simulink model "assignment2_group12"  (R2021a)
settings: Solver=FixedStepAuto  StartTime=0.0  StopTime=10.0  FixedStep=1e-3  RelTol=1e-3  EnableMultiTasking=on
undefined symbols (not defined in the file): A0, A1, D0, D1, D10, D11, D12, D13, D2, D3, D4, D5, D6, D7, D8, D9, PTA0, PTA1, PTA2, PTB2, PTB23, PTB3, PTB9, PTC16, PTC17, PTC2, PTC3, PTC4, PTD0, PTD1, PTD2, PTD3
libraries: frdmk64flib x19, etargetslib x18, dspstat3 x1
settings Model: ExtModeTrigDuration=5  Creator=shoghisama  LastModifiedBy=shoghisama
settings OptimizationCC: EnhancedBackFolding=on  PassReuseOutputArgsAs=Individual arguments  ZeroExternalMemoryAtStartup=off  ZeroInternalMemoryAtStartup=off  MaxStackSize=64  OptimizeBlockOrder=speed  DifferentSizesBufferReuse=on  OptimizationCustomize=off  EfficientTunableParamExpr=on
settings DebuggingCC: ParameterTunabilityLossMsg=error
settings HardwareCC: ProdBitPerPointer=32  ProdBitPerSizeT=32  ProdBitPerPtrDiffT=32  ProdLargestAtomicInteger=Long  ProdLargestAtomicFloat=Double  ProdWordSize=32  ProdHWDeviceType=ARM Compatible->ARM Cortex
settings SFSimCC: MATLABDynamicMemAlloc=off
settings RTWCC: SystemTargetFile=ert.tlc  HardwareBoard=NXP FRDM-K64F  TLCOptions="-aInlineSetEventsForThisBaseRateFcn=TLC_FALSE -aSuppressMultiTaskScheduler=TLC_FALSE  -aRateBasedStepFcn=0"  TemplateMakefile=ert_default_tmf  Toolchain=GNU Tools for ARM Embedded Processors
settings CodeAppCC: ForceParamTrailComments=on  IgnoreCustomStorageClasses=off  OperatorAnnotations=on  SimulinkDataObjDesc=on  SFDataObjDesc=on  InsertBlockDesc=on
settings ERTTargetCC: ExtModeTransport=4  ExtModeMexFile=sendToCommService

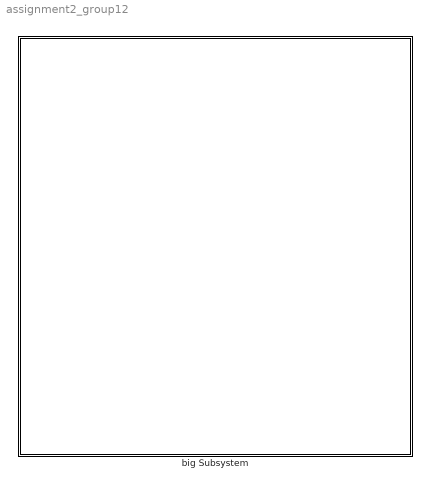
== system assignment2_group12 ==
  big Subsystem : Subsystem

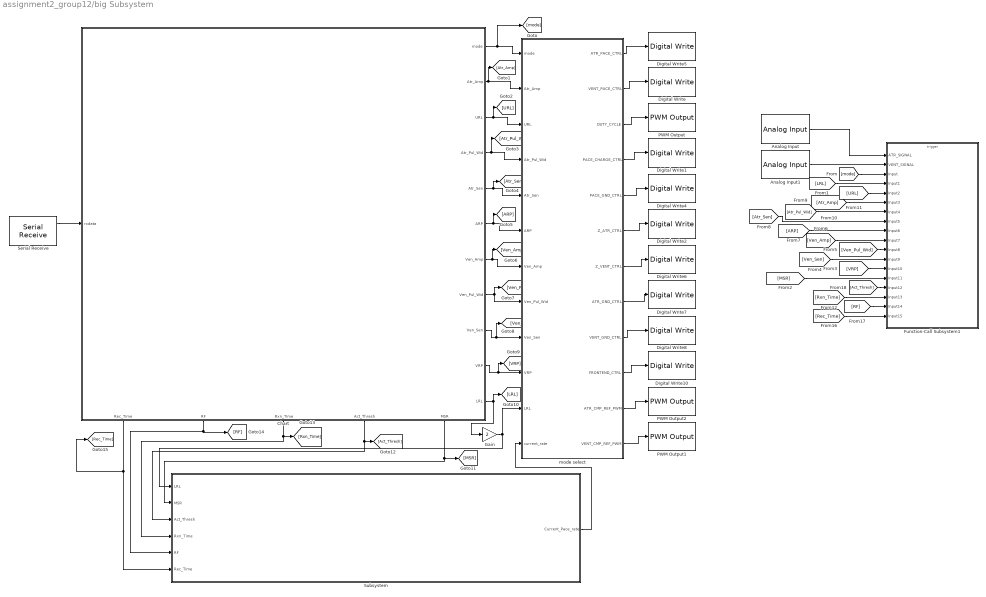
== system assignment2_group12/big Subsystem ==
  Analog Input : frdmk64flib/Analog Input  Whichpin=PTB2 (A0)  SampleTime=-1
  Analog Input1 : frdmk64flib/Analog Input  Whichpin=PTB3 (A1)  SampleTime=-1
  Chart : Stateflow chart  TreatAsAtomicUnit=on
      settings: PortSchema="{\"entries\":[{\"content\":{\"sides\":[{\"content\":{\"connectorIds\":[\"In1\"]},\"type\":\"ConnectorPlacement.EquallySpacedRectSide\",\"uuid\":\"029204fe-544c-471c-b678-20eb9ec2f0de\"},{\"content\":{\"connectorIds\":[\"Out16\",\"Out2\",\"Out3\",\"Out4\",\"Out5\",\"Out6\",\"Out7\",\"Out8\",\"Out9\",\"Out10\",\"Out1\"],\"side\":\"RIGHT\"},\"type\":\"ConnectorPlacement.EquallySpacedRectSide\",\"uuid\":\"7eca2d38-9628-43b8-9613-7fbfe5c4b303\"},{\"content\":{\"connectorIds\":[],\"side\":\"TOP\"},\"type\":\"ConnectorPlacement.EquallySpacedRectSide\",\"uuid\":\"096b792e-b126-4483-96fc-02dd5bb2fe66\"},{\"content\":{\"connectorIds\":[\"Out15\",\"Out14\",\"Out13\",\"Out12\",\"Out11\"],\"side\":\"BOTTOM\"},\"type\":\"ConnectorPlacement.EquallySpacedRectSide\",\"uuid\":\"986cb6f9-09d3-4d0e-abe9-ddef6787962a\"}]},\"type\":\"ConnectorPlacement.EquallySpacedConnector\",\"uuid\":\"f90ba696-ad08-4385-b69c-5e6e3d9fa11d\"}],\"packageUris\":[\"http://schema.mathworks.com/mf0/Connector/R2020b\"],\"version\":\"1.0\"}"
  Digital Write : frdmk64flib/Digital Write  Whichpin=PTC4 (D9)
  Digital Write1 : frdmk64flib/Digital Write  Whichpin=PTB9 (D2)
  Digital Write10 : frdmk64flib/Digital Write  Whichpin=PTD1 (D13)
  Digital Write2 : frdmk64flib/Digital Write  Whichpin=PTB23 (D4)
  Digital Write4 : frdmk64flib/Digital Write  Whichpin=PTD0 (D10)
  Digital Write5 : frdmk64flib/Digital Write  Whichpin=PTA0 (D8)
  Digital Write6 : frdmk64flib/Digital Write  Whichpin=PTC3 (D7)
  Digital Write7 : frdmk64flib/Digital Write  Whichpin=PTD2 (D11)
  Digital Write8 : frdmk64flib/Digital Write  Whichpin=PTD3 (D12)
  Function-Call Subsystem1 : Subsystem  TreatAsAtomicUnit=on
  Gain : Gain  Gain=2  OutDataTypeStr=double
  PWM Output : frdmk64flib/PWM Output  Whichpin=PTA2 (D5)  InitialFrequency=2000  InitialDutyCycle=0
  PWM Output1 : frdmk64flib/PWM Output  Whichpin=PTA1 (D3)  InitialFrequency=2000  InitialDutyCycle=0
  PWM Output2 : frdmk64flib/PWM Output  Whichpin=PTC2 (D6)  InitialFrequency=2000  InitialDutyCycle=0
  Serial Receive : frdmk64flib/Serial Receive  SCIModule=0  Baudrate=uint32(9600)  Parity=None  StopBits=1  HardwareFlowControl=None  ByteOrder=LittleEndian  DataType=uint8  DataLength=123  BlockingMode=off  OutputStatus=on  SampleTime=-1
  Subsystem : Subsystem
  mode select : Subsystem
  wires:
  Chart/4(Atr_Pul_Wid) -> [Atr_Pul_Wid], mode select/4(Atr_Pul_Wid)
  Chart/5(Atr_Sen) -> [Atr_Sen], mode select/5(Atr_Sen)
  mode select/8(ATR_GND_CTRL) -> Digital Write7/1
  mode select/4(PACE_CHARGE_CTRL) -> Digital Write1/1
  mode select/1(ATR_PACE_CTRL) -> Digital Write5/1
  mode select/2(VENT_PACE_CTRL) -> Digital Write/1
  mode select/5(PACE_GND_CTRL) -> Digital Write4/1
  mode select/6(Z_ATR_CTRL) -> Digital Write2/1
  mode select/10(FRONTEND_CTRL) -> Digital Write10/1
  mode select/7(Z_VENT_CTRL) -> Digital Write6/1
  mode select/3(DUTY_CYCLE) -> PWM Output/1
  mode select/9(VENT_GND_CTRL) -> Digital Write8/1
  mode select/12(VENT_CMP_REF_PWM) -> PWM Output1/1
  mode select/11(ATR_CMP_REF_PWM) -> PWM Output2/1
  Chart/2(Atr_Amp) -> mode select/2(Atr_Amp), [Atr_Amp]
  Chart/11(MSR) -> [MSR], Subsystem/2(MSR)
  Chart/12(Act_Thresh) -> [Act_Thresh], Subsystem/3(Act_Thresh)
  Chart/13(Rxn_Time) -> Subsystem/4(Rxn_Time), [Rxn_Time]
  Chart/14(RF) -> [RF], Subsystem/5(RF)
  Chart/15(Rec_Time) -> [Rec_Time], Subsystem/6(Rec_Time)
  Serial Receive/1 -> Chart/1(rxdata)
  Chart/6(ARP) -> [ARP], mode select/6(ARP)
  Chart/7(Ven_Amp) -> [Ven_Amp], mode select/7(Ven_Amp)
  Chart/10(VRP) -> [VRP], mode select/10(VRP)
  Chart/9(Ven_Sen) -> [Ven_Sen], mode select/9(Ven_Sen)
  Chart/8(Ven_Pul_Wid) -> mode select/8(Ven_Pul_Wid), [Ven_Pul_Wid]
  Chart/3(URL) -> [URL], mode select/3(URL)
  Subsystem/1(Current_Pace_rate) -> mode select/12(current_rate)
  Gain/1 -> mode select/11(LRL), Subsystem/1(LRL)
  Chart/16(mode) -> [mode], mode select/1(mode)
  Chart/1(LRL) -> Gain/1, [LRL]
  [ARP] -> Function-Call Subsystem1/9(Input6)
  [Rec_Time] -> Function-Call Subsystem1/18(Input15)
  [Ven_Pul_Wid] -> Function-Call Subsystem1/11(Input8)
  [URL] -> Function-Call Subsystem1/5(Input2)
  Analog Input/1 -> Function-Call Subsystem1/1(ATR_SIGNAL)
  [Atr_Sen] -> Function-Call Subsystem1/8(Input5)
  [VRP] -> Function-Call Subsystem1/13(Input10)
  [Ven_Sen] -> Function-Call Subsystem1/12(Input9)
  [LRL] -> Function-Call Subsystem1/4(Input1)
  [MSR] -> Function-Call Subsystem1/14(Input11)
  [Ven_Amp] -> Function-Call Subsystem1/10(Input7)
  [Atr_Pul_Wid] -> Function-Call Subsystem1/7(Input4)
  Analog Input1/1 -> Function-Call Subsystem1/2(VENT_SIGNAL)
  [Rxn_Time] -> Function-Call Subsystem1/16(Input13)
  [RF] -> Function-Call Subsystem1/17(Input14)
  [mode] -> Function-Call Subsystem1/3(Input)
  [Atr_Amp] -> Function-Call Subsystem1/6(Input3)
  [Act_Thresh] -> Function-Call Subsystem1/15(Input12)

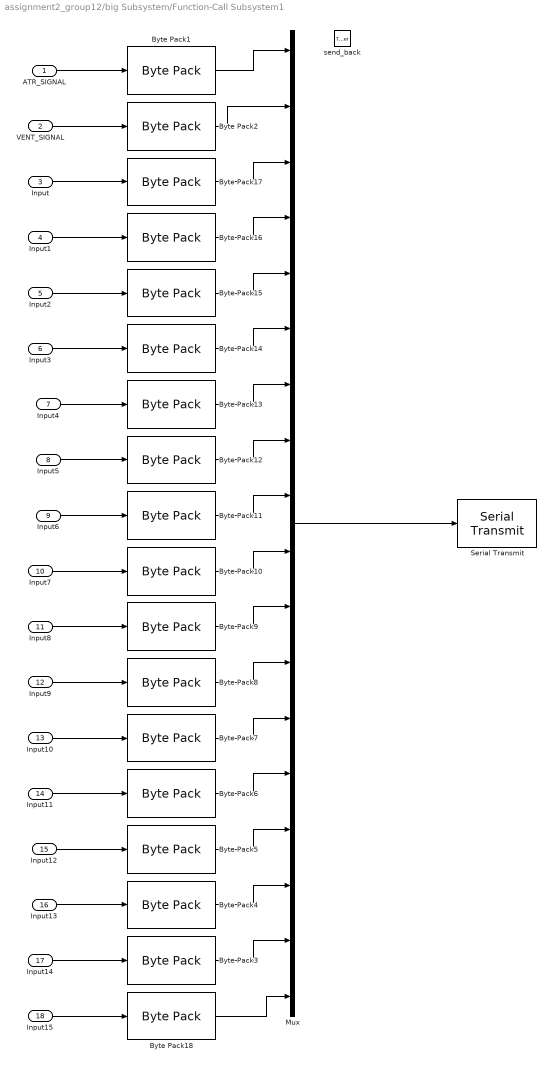
== system assignment2_group12/big Subsystem/Function-Call Subsystem1 ==
  ATR_SIGNAL : Inport  OutDataTypeStr=double
  VENT_SIGNAL : Inport  Port=2  OutDataTypeStr=double
  Input : Inport  Port=3
  Input1 : Inport  Port=4
  Input2 : Inport  Port=5
  Input3 : Inport  Port=6
  Input4 : Inport  Port=7
  Input5 : Inport  Port=8
  Input6 : Inport  Port=9
  Input7 : Inport  Port=10
  Input8 : Inport  Port=11
  Input9 : Inport  Port=12
  Input10 : Inport  Port=13
  Input11 : Inport  Port=14
  Input12 : Inport  Port=15
  Input13 : Inport  Port=16
  Input14 : Inport  Port=17
  Input15 : Inport  Port=18
  send_back : TriggerPort  TriggerType=function-call  IsSimulinkFunction=on  FunctionName=send_back  VariantControl=Variant
  Byte Pack{1..16,18} (17 alike) : etargetslib/Byte Pack  datatypes={'double'}  byteAlign=1
  Byte Pack17 : etargetslib/Byte Pack  datatypes={'uint8'}  byteAlign=1
  Mux : Mux  Inputs=18
  Serial Transmit : frdmk64flib/Serial Transmit  SCIModule=0  Baudrate=uint32(9600)  Parity=None  StopBits=1  HardwareFlowControl=None  ByteOrder=LittleEndian  BlockingMode=on  OutputStatus=off
  wires:
  Mux/1 -> Serial Transmit/1
  ATR_SIGNAL/1 -> Byte Pack1/1
  Byte Pack1/1 -> Mux/1
  VENT_SIGNAL/1 -> Byte Pack2/1
  Byte Pack2/1 -> Mux/2
  Input/1 -> Byte Pack17/1
  Input1/1 -> Byte Pack16/1
  Input2/1 -> Byte Pack15/1
  Input3/1 -> Byte Pack14/1
  Input4/1 -> Byte Pack13/1
  Input5/1 -> Byte Pack12/1
  Input6/1 -> Byte Pack11/1
  Input7/1 -> Byte Pack10/1
  Input8/1 -> Byte Pack9/1
  Input9/1 -> Byte Pack8/1
  Input13/1 -> Byte Pack4/1
  Input14/1 -> Byte Pack3/1
  Input12/1 -> Byte Pack5/1
  Input11/1 -> Byte Pack6/1
  Input10/1 -> Byte Pack7/1
  Byte Pack17/1 -> Mux/3
  Byte Pack16/1 -> Mux/4
  Byte Pack15/1 -> Mux/5
  Byte Pack14/1 -> Mux/6
  Byte Pack13/1 -> Mux/7
  Byte Pack12/1 -> Mux/8
  Byte Pack11/1 -> Mux/9
  Byte Pack10/1 -> Mux/10
  Byte Pack9/1 -> Mux/11
  Byte Pack8/1 -> Mux/12
  Byte Pack7/1 -> Mux/13
  Byte Pack6/1 -> Mux/14
  Byte Pack5/1 -> Mux/15
  Byte Pack4/1 -> Mux/16
  Byte Pack3/1 -> Mux/17
  Input15/1 -> Byte Pack18/1
  Byte Pack18/1 -> Mux/18

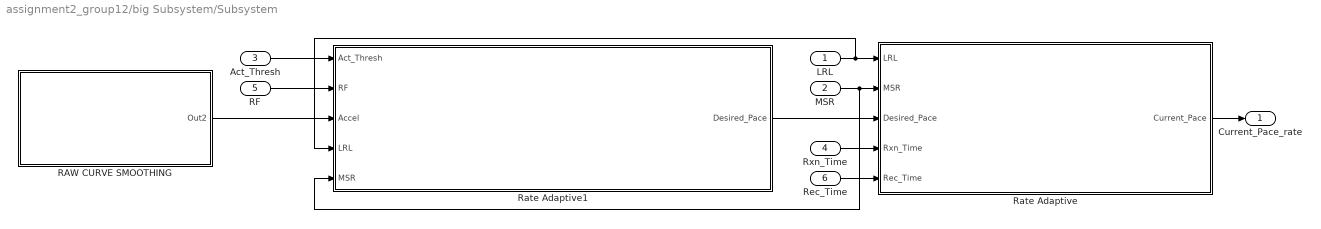
== system assignment2_group12/big Subsystem/Subsystem ==
  LRL : Inport
  MSR : Inport  Port=2
  Act_Thresh : Inport  Port=3
  Rxn_Time : Inport  Port=4
  RF : Inport  Port=5
  Rec_Time : Inport  Port=6
  "RAW CURVE SMOOTHING " : Subsystem
  Rate Adaptive : Stateflow chart  TreatAsAtomicUnit=on
      settings: PortSchema="{\"entries\":[{\"content\":{\"sides\":[{\"content\":{\"connectorIds\":[\"In2\",\"In3\",\"In1\",\"In4\",\"In5\"]},\"type\":\"ConnectorPlacement.EquallySpacedRectSide\",\"uuid\":\"2415e76f-d31e-4d4d-9cdd-20c640b682ec\"},{\"content\":{\"connectorIds\":[\"Out1\"],\"side\":\"RIGHT\"},\"type\":\"ConnectorPlacement.EquallySpacedRectSide\",\"uuid\":\"7e1eacd0-064b-4f4a-b34f-1b700ef5f1aa\"},{\"content\":{\"connectorIds\":[],\"side\":\"TOP\"},\"type\":\"ConnectorPlacement.EquallySpacedRectSide\",\"uuid\":\"9000ba44-c9a9-4586-8c67-e4f8d554e570\"}]},\"type\":\"ConnectorPlacement.EquallySpacedConnector\",\"uuid\":\"f24a2368-4906-4838-a1d8-28d9fed4dceb\"}],\"packageUris\":[\"http://schema.mathworks.com/mf0/Connector/R2020b\"],\"version\":\"1.0\"}"
  Rate Adaptive1 : Stateflow chart  TreatAsAtomicUnit=on
  Current_Pace_rate : Outport
  wires:
  Rate Adaptive1/1(Desired_Pace) -> Rate Adaptive/1(Desired_Pace)
  RF/1 -> Rate Adaptive1/2(RF)
  Act_Thresh/1 -> Rate Adaptive1/1(Act_Thresh)
  "RAW CURVE SMOOTHING "/1(Out2) -> Rate Adaptive1/3(Accel)
  Rec_Time/1 -> Rate Adaptive/5(Rec_Time)
  Rxn_Time/1 -> Rate Adaptive/4(Rxn_Time)
  MSR/1 -> Rate Adaptive1/5(MSR), Rate Adaptive/3(MSR)
  LRL/1 -> Rate Adaptive1/4(LRL), Rate Adaptive/2(LRL)
  Rate Adaptive/1(Current_Pace) -> Current_Pace_rate/1

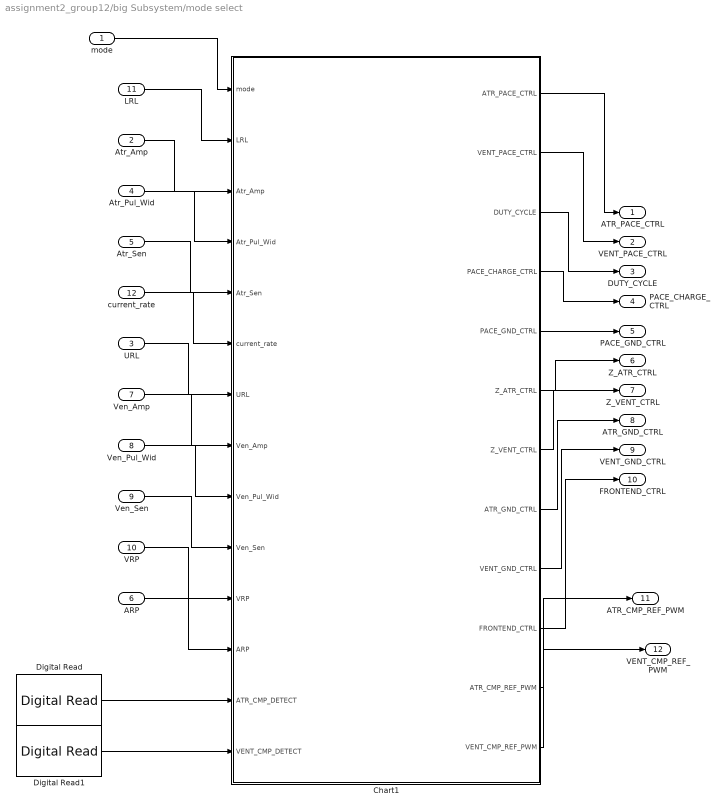
== system assignment2_group12/big Subsystem/mode select ==
  mode : Inport
  Atr_Amp : Inport  Port=2  OutDataTypeStr=double
  URL : Inport  Port=3
  Atr_Pul_Wid : Inport  Port=4
  Atr_Sen : Inport  Port=5
  ARP : Inport  Port=6
  Ven_Amp : Inport  Port=7
  Ven_Pul_Wid : Inport  Port=8
  Ven_Sen : Inport  Port=9
  VRP : Inport  Port=10
  LRL : Inport  Port=11  OutDataTypeStr=double
  current_rate : Inport  Port=12
  Chart1 : Stateflow chart  TreatAsAtomicUnit=on
      settings: PortSchema="{\"entries\":[{\"content\":{\"sides\":[{\"content\":{\"connectorIds\":[\"In13\",\"In1\",\"In2\",\"In3\",\"In6\",\"In7\",\"In8\",\"In9\",\"In10\",\"In11\",\"In12\",\"In14\",\"In4\",\"In5\"]},\"type\":\"ConnectorPlacement.EquallySpacedRectSide\",\"uuid\":\"48eae28e-eb31-49cd-a267-63fca9261c17\"},{\"content\":{\"connectorIds\":[\"Out1\",\"Out2\",\"Out3\",\"Out4\",\"Out5\",\"Out6\",\"Out7\",\"Out8\",\"Out9\",\"Out10\",\"Out11\",\"Out12\"],\"side\":\"RIGHT\"},\"type\":\"ConnectorPlacement.EquallySpacedRectSide\",\"uuid\":\"b92b5989-7079-44f9-b40b-bd28ed96be33\"},{\"content\":{\"connectorIds\":[],\"side\":\"TOP\"},\"type\":\"ConnectorPlacement.EquallySpacedRectSide\",\"uuid\":\"1f742a6a-0314-45aa-83af-1ea6ddab1409\"}]},\"type\":\"ConnectorPlacement.EquallySpacedConnector\",\"uuid\":\"9519d4d5-861f-4553-8ea3-55a3fc1f944b\"}],\"packageUris\":[\"http://schema.mathworks.com/mf0/Connector/R2020b\"],\"version\":\"1.0\"}"
  Digital Read : frdmk64flib/Digital Read  Whichpin=PTC16 (D0)  SampleTime=-1
  Digital Read1 : frdmk64flib/Digital Read  Whichpin=PTC17 (D1)  SampleTime=-1
  ATR_PACE_CTRL : Outport
  VENT_PACE_CTRL : Outport  Port=2
  DUTY_CYCLE : Outport  Port=3
  PACE_CHARGE_CTRL : Outport  Port=4
  PACE_GND_CTRL : Outport  Port=5
  Z_ATR_CTRL : Outport  Port=6
  Z_VENT_CTRL : Outport  Port=7
  ATR_GND_CTRL : Outport  Port=8
  VENT_GND_CTRL : Outport  Port=9
  FRONTEND_CTRL : Outport  Port=10
  ATR_CMP_REF_PWM : Outport  Port=11
  VENT_CMP_REF_PWM : Outport  Port=12
  wires:
  Atr_Amp/1 -> Chart1/2(Atr_Amp)
  Atr_Pul_Wid/1 -> Chart1/3(Atr_Pul_Wid)
  ARP/1 -> Chart1/14(ARP)
  LRL/1 -> Chart1/1(LRL)
  Digital Read/1 -> Chart1/4(ATR_CMP_DETECT)
  Digital Read1/1 -> Chart1/5(VENT_CMP_DETECT)
  mode/1 -> Chart1/13(mode)
  Chart1/7(Z_VENT_CTRL) -> Z_VENT_CTRL/1
  Chart1/9(VENT_GND_CTRL) -> VENT_GND_CTRL/1
  Chart1/4(PACE_CHARGE_CTRL) -> PACE_CHARGE_CTRL/1
  Chart1/2(VENT_PACE_CTRL) -> VENT_PACE_CTRL/1
  Chart1/8(ATR_GND_CTRL) -> ATR_GND_CTRL/1
  Chart1/6(Z_ATR_CTRL) -> Z_ATR_CTRL/1
  Chart1/5(PACE_GND_CTRL) -> PACE_GND_CTRL/1
  Chart1/1(ATR_PACE_CTRL) -> ATR_PACE_CTRL/1
  Chart1/3(DUTY_CYCLE) -> DUTY_CYCLE/1
  Chart1/10(FRONTEND_CTRL) -> FRONTEND_CTRL/1
  Chart1/11(ATR_CMP_REF_PWM) -> ATR_CMP_REF_PWM/1
  Chart1/12(VENT_CMP_REF_PWM) -> VENT_CMP_REF_PWM/1
  Atr_Sen/1 -> Chart1/6(Atr_Sen)
  current_rate/1 -> Chart1/7(current_rate)
  URL/1 -> Chart1/8(URL)
  Ven_Amp/1 -> Chart1/9(Ven_Amp)
  Ven_Pul_Wid/1 -> Chart1/10(Ven_Pul_Wid)
  VRP/1 -> Chart1/12(VRP)
  Ven_Sen/1 -> Chart1/11(Ven_Sen)

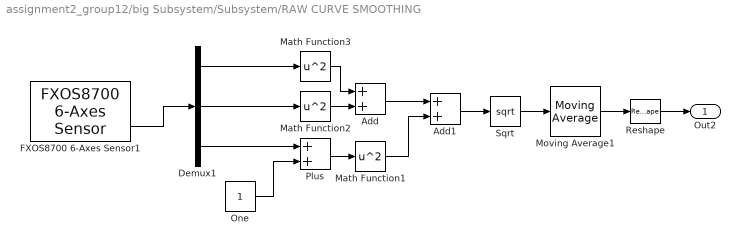
== system assignment2_group12/big Subsystem/Subsystem/RAW CURVE SMOOTHING  ==
  Add : Sum
  Add1 : Sum
  Demux1 : Demux  Outputs=3
  FXOS8700 6-Axes Sensor1 : frdmk64flib/FXOS8700 6-Axes Sensor  Activesensor=Accelerometer and Magnetometer  ODR=800Hz  HybridODR=400Hz  Accelfullrange=-8g to +8g  SampleTime=-1
  Math Function1 : Math  Operator=square  SaturateOnIntegerOverflow=on
  Math Function2 : Math  Operator=square  SaturateOnIntegerOverflow=on
  Math Function3 : Math  Operator=square  SaturateOnIntegerOverflow=on
  Moving Average1 : dspstat3/Moving Average  Method=Sliding window  ForgettingFactorPort=off  SpecifyWindowLength=on  WindowLength=30  ForgettingFactor=0.9  SimulateUsing=Code generation
  One : Constant  OutDataTypeStr=Inherit: Inherit via back propagation
  Plus : Sum
  Reshape : Reshape
  Sqrt : Sqrt  SaturateOnIntegerOverflow=on
  Out2 : Outport
  wires:
  Demux1/1 -> Math Function3/1
  Add/1 -> Add1/1
  FXOS8700 6-Axes Sensor1/2 -> Demux1/1
  Sqrt/1 -> Moving Average1/1
  Demux1/2 -> Math Function2/1
  Add1/1 -> Sqrt/1
  Math Function3/1 -> Add/1
  Math Function1/1 -> Add1/2
  Math Function2/1 -> Add/2
  One/1 -> Plus/2
  Demux1/3 -> Plus/1
  Plus/1 -> Math Function1/1
  Moving Average1/1 -> Reshape/1
  Reshape/1 -> Out2/1

== stateflow chart assignment2_group12/big Subsystem/mode select/Chart1 ==
  state CHARGING_DISCHARGING
    entry:
    ATR_PACE_CTRL=false
    VENT_PACE_CTRL=false
    DUTY_CYCLE=Atr_Amp/0.05
    PACE_CHARGE_CTRL=true
    PACE_GND_CTRL=true
    Z_ATR_CTRL=false
    Z_VENT_CTRL=false
    ATR_GND_CTRL=true
    VENT_GND_CTRL=false
  state ATRIAL_PACING
    entry:
    PACE_CHARGE_CTRL=false
    PACE_GND_CTRL=true
    ATR_PACE_CTRL=true
    ATR_GND_CTRL=false
    Z_ATR_CTRL=false
    Z_VENT_CTRL=false
    VENT_GND_CTRL=false
    VENT_PACE_CTRL=false
  state CHARGING_DISCHARGING3
    entry:
    ATR_PACE_CTRL=false
    VENT_PACE_CTRL=false
    DUTY_CYCLE=Atr_Amp/0.05
    PACE_CHARGE_CTRL=true
    PACE_GND_CTRL=true
    Z_ATR_CTRL=false
    Z_VENT_CTRL=false
    ATR_GND_CTRL=true
    VENT_GND_CTRL=false
  state ATRIAL_PACING4
    entry:
    PACE_CHARGE_CTRL=false
    PACE_GND_CTRL=true
    ATR_PACE_CTRL=true
    ATR_GND_CTRL=false
    Z_ATR_CTRL=false
    Z_VENT_CTRL=false
    VENT_GND_CTRL=false
    VENT_PACE_CTRL=false
  state CHARGING_DISCHARGING1
    entry:
    ATR_PACE_CTRL=false
    VENT_PACE_CTRL=false
    DUTY_CYCLE=Ven_Amp/0.05
    PACE_CHARGE_CTRL=true
    PACE_GND_CTRL=true
    Z_ATR_CTRL=false
    Z_VENT_CTRL=false
    ATR_GND_CTRL=false
    VENT_GND_CTRL=true
  state VENTRICULAR_PACING
    entry:
    PACE_CHARGE_CTRL=false
    PACE_GND_CTRL=true
    ATR_PACE_CTRL=false
    ATR_GND_CTRL=false
    Z_ATR_CTRL=false
    Z_VENT_CTRL=false
    VENT_GND_CTRL=false
    VENT_PACE_CTRL=true
  state CHARGING_DISCHARGING2
    entry:
    ATR_PACE_CTRL=false
    VENT_PACE_CTRL=false
    DUTY_CYCLE=Ven_Amp/0.05
    PACE_CHARGE_CTRL=true
    PACE_GND_CTRL=true
    Z_ATR_CTRL=false
    Z_VENT_CTRL=false
    ATR_GND_CTRL=false
    VENT_GND_CTRL=true
  state VENTRICULAR_PACING3
    entry:
    PACE_CHARGE_CTRL=false
    PACE_GND_CTRL=true
    ATR_PACE_CTRL=false
    ATR_GND_CTRL=false
    Z_ATR_CTRL=false
    Z_VENT_CTRL=false
    VENT_GND_CTRL=false
    VENT_PACE_CTRL=true
  state iniitial
  state CHARGING_DISCHARGING_SENSING
    entry:
    ATR_PACE_CTRL=false
    VENT_PACE_CTRL=false
    DUTY_CYCLE=Atr_Amp/0.05
    PACE_CHARGE_CTRL=true
    PACE_GND_CTRL=true
    Z_ATR_CTRL=false
    Z_VENT_CTRL=false
    ATR_GND_CTRL=true
    VENT_GND_CTRL=false
    FRONTEND_CTRL=true
    ATR_CMP_REF_PWM=Atr_Sen/0.05
    (junction 35) -> (junction 39) : [ATR_CMP_DETECT==true]
    CHARGING_DISCHARGING_SENSING -> (junction 35) [order 1] : [after(ARP,msec)]
    (junction 39) -> (junction 40) : {Sensed=true}
  state ATRIAL_PACING1
    entry:
    PACE_CHARGE_CTRL=false
    PACE_GND_CTRL=true
    ATR_PACE_CTRL=true
    ATR_GND_CTRL=false
    Z_ATR_CTRL=false
    Z_VENT_CTRL=false
    VENT_GND_CTRL=false
    VENT_PACE_CTRL=false
    Sensed=true
  state CHARGING_DISCHARGING_SENSING2
    entry:
    ATR_PACE_CTRL=false
    VENT_PACE_CTRL=false
    DUTY_CYCLE=Atr_Amp/0.05
    PACE_CHARGE_CTRL=true
    PACE_GND_CTRL=true
    Z_ATR_CTRL=false
    Z_VENT_CTRL=false
    ATR_GND_CTRL=true
    VENT_GND_CTRL=false
    FRONTEND_CTRL=true
    ATR_CMP_REF_PWM=Atr_Sen/0.05
    CHARGING_DISCHARGING_SENSING2 -> (junction 136) [order 1] : [after(ARP,msec)]
    (junction 136) -> (junction 138) : [ATR_CMP_DETECT==true]
    (junction 138) -> (junction 134) : {Sensed=true}
  state ATRIAL_PACING3
    entry:
    PACE_CHARGE_CTRL=false
    PACE_GND_CTRL=true
    ATR_PACE_CTRL=true
    ATR_GND_CTRL=false
    Z_ATR_CTRL=false
    Z_VENT_CTRL=false
    VENT_GND_CTRL=false
    VENT_PACE_CTRL=false
    Sensed=true
  state CONDITION_CHECK
    entry:
  state CONDITION_CHECK2
    entry:
  state CHARGING_DISCHARGING_SENSING1
    entry:
    ATR_PACE_CTRL=false
    VENT_PACE_CTRL=false
    DUTY_CYCLE=Ven_Amp/0.05
    PACE_CHARGE_CTRL=true
    PACE_GND_CTRL=true
    Z_ATR_CTRL=false
    Z_VENT_CTRL=false
    ATR_GND_CTRL=false
    VENT_GND_CTRL=true
    FRONTEND_CTRL=true
    VENT_CMP_REF_PWM=Ven_Sen/0.05
    (junction 49) -> (junction 53) : [VENT_CMP_DETECT==true]
    CHARGING_DISCHARGING_SENSING1 -> (junction 49) [order 1] : [after(VRP,msec)]
    (junction 53) -> (junction 51) : {Sensed=true}
  state VENTRICULAR_PACING2
    entry:
    PACE_CHARGE_CTRL=false
    PACE_GND_CTRL=true
    ATR_PACE_CTRL=false
    ATR_GND_CTRL=false
    Z_ATR_CTRL=false
    Z_VENT_CTRL=false
    VENT_GND_CTRL=false
    VENT_PACE_CTRL=true
    Sensed=true
  state CHARGING_DISCHARGING_SENSING3
    entry:
    ATR_PACE_CTRL=false
    VENT_PACE_CTRL=false
    DUTY_CYCLE=Ven_Amp/0.05
    PACE_CHARGE_CTRL=true
    PACE_GND_CTRL=true
    Z_ATR_CTRL=false
    Z_VENT_CTRL=false
    ATR_GND_CTRL=false
    VENT_GND_CTRL=true
    FRONTEND_CTRL=true
    VENT_CMP_REF_PWM=Ven_Sen/0.05
    CHARGING_DISCHARGING_SENSING3 -> (junction 139) [order 1] : [after(VRP,msec)]
    (junction 144) -> (junction 142) : {Sensed=true}
    (junction 139) -> (junction 144) : [VENT_CMP_DETECT==true]
  state VENTRICULAR_PACING4
    entry:
    PACE_CHARGE_CTRL=false
    PACE_GND_CTRL=true
    ATR_PACE_CTRL=false
    ATR_GND_CTRL=false
    Z_ATR_CTRL=false
    Z_VENT_CTRL=false
    VENT_GND_CTRL=false
    VENT_PACE_CTRL=true
    Sensed=true
  state CONDITION_CHECK1
  state CONDITION_CHECK3
  iniitial -> CHARGING_DISCHARGING [order 1] : [mode == 1]
  ATRIAL_PACING -> CHARGING_DISCHARGING : [after(Atr_Pul_Wid,msec)]
  CHARGING_DISCHARGING -> iniitial [order 2] : [mode ~= 1]
  CHARGING_DISCHARGING3 -> ATRIAL_PACING4 [order 2] : [after(((60000-(current_rate*Atr_Pul_Wid))/current_rate),msec)]
  iniitial -> CHARGING_DISCHARGING3 [order 6] : [mode == 5]
  CHARGING_DISCHARGING -> ATRIAL_PACING [order 1] : [after(((60000-(LRL*Atr_Pul_Wid))/LRL),msec)]
  CHARGING_DISCHARGING3 -> iniitial [order 1] : [mode ~= 5]
  ATRIAL_PACING4 -> CHARGING_DISCHARGING3 : [after(Atr_Pul_Wid,msec)]
  iniitial -> CHARGING_DISCHARGING1 [order 2] : [mode == 2]
  VENTRICULAR_PACING -> CHARGING_DISCHARGING1 : [after(Ven_Pul_Wid,msec)]
  CHARGING_DISCHARGING2 -> VENTRICULAR_PACING3 [order 2] : [after(((60000-(current_rate*Ven_Pul_Wid))/current_rate),msec)]
  CHARGING_DISCHARGING1 -> iniitial [order 2] : [mode ~= 2]
  iniitial -> CHARGING_DISCHARGING2 [order 7] : [mode == 6]
  CHARGING_DISCHARGING1 -> VENTRICULAR_PACING [order 1] : [after(((60000-(LRL*Ven_Pul_Wid))/LRL),msec)]
  (default) -> iniitial
  VENTRICULAR_PACING3 -> CHARGING_DISCHARGING2 : [after(Ven_Pul_Wid,msec)]
  CHARGING_DISCHARGING2 -> iniitial [order 1] : [mode ~= 6]
  iniitial -> CHARGING_DISCHARGING_SENSING [order 3] : [mode == 3]
  CONDITION_CHECK -> ATRIAL_PACING1 [order 1] : [Sensed==false]
  CHARGING_DISCHARGING_SENSING -> CONDITION_CHECK [order 1] : [after(((60000-(LRL*Atr_Pul_Wid))/LRL),msec)]
  iniitial -> CHARGING_DISCHARGING_SENSING2 [order 8] : [mode == 7]
  ATRIAL_PACING1 -> CONDITION_CHECK : [after(Atr_Pul_Wid,msec)]
  CONDITION_CHECK2 -> CHARGING_DISCHARGING_SENSING2 [order 2] : {Sensed=false}
  CHARGING_DISCHARGING_SENSING -> iniitial [order 2] : [mode~=3]
  CONDITION_CHECK -> CHARGING_DISCHARGING_SENSING [order 2] : {Sensed=false}
  CHARGING_DISCHARGING_SENSING2 -> iniitial [order 1] : [mode ~= 7]
  ATRIAL_PACING3 -> CONDITION_CHECK2 : [after(Atr_Pul_Wid,msec)]
  CHARGING_DISCHARGING_SENSING2 -> CONDITION_CHECK2 [order 2] : [after(((60000-(current_rate*Atr_Pul_Wid))/current_rate),msec)]
  CONDITION_CHECK2 -> ATRIAL_PACING3 [order 1] : [Sensed==false]
  iniitial -> CHARGING_DISCHARGING_SENSING3 [order 5] : [mode == 8]
  iniitial -> CHARGING_DISCHARGING_SENSING1 [order 4] : [mode == 4]
  CHARGING_DISCHARGING_SENSING3 -> iniitial [order 1] : [mode ~= 8]
  CHARGING_DISCHARGING_SENSING1 -> iniitial [order 2] : [mode ~= 4]
  CONDITION_CHECK1 -> VENTRICULAR_PACING2 [order 1] : [Sensed==false]
  CHARGING_DISCHARGING_SENSING1 -> CONDITION_CHECK1 [order 1] : [after(((60000-(LRL*Ven_Pul_Wid))/LRL),msec)]
  VENTRICULAR_PACING2 -> CONDITION_CHECK1 : [after(Ven_Pul_Wid,msec)]
  CONDITION_CHECK1 -> CHARGING_DISCHARGING_SENSING1 [order 2] : {Sensed=false}
  CONDITION_CHECK3 -> CHARGING_DISCHARGING_SENSING3 [order 2] : {Sensed=false}
  VENTRICULAR_PACING4 -> CONDITION_CHECK3 : [after(Ven_Pul_Wid,msec)]
  CHARGING_DISCHARGING_SENSING3 -> CONDITION_CHECK3 [order 2] : [after(((60000-(current_rate*Ven_Pul_Wid))/current_rate),msec)]
  CONDITION_CHECK3 -> VENTRICULAR_PACING4 [order 1] : [Sensed==false]
  data: LRL input double; Atr_Amp input double; Atr_Pul_Wid input double; ATR_PACE_CTRL output boolean; VENT_PACE_CTRL output boolean; DUTY_CYCLE output double; PACE_CHARGE_CTRL output boolean; PACE_GND_CTRL output boolean; Z_ATR_CTRL output boolean; Z_VENT_CTRL output boolean; ATR_GND_CTRL output boolean; VENT_GND_CTRL output boolean; ATR_CMP_DETECT input boolean; VENT_CMP_DETECT input boolean; FRONTEND_CTRL output boolean; ATR_CMP_REF_PWM output double; VENT_CMP_REF_PWM output double; Atr_Sen input double; Sensed local boolean =false; current_rate input double; URL input double; Ven_Amp input double; Ven_Pul_Wid input double; Ven_Sen input double; VRP input double; mode input uint8; ARP input double

== stateflow chart assignment2_group12/big Subsystem/Subsystem/Rate Adaptive1 ==
  state check2
    entry:
    Desired_Pace = Desired_Pace1
  state check
    entry:
    Desired_Pace1 = m_slope*RF*Act_Lvl+LRL
  state init
    entry:
    Act_Thresh_Max = 7
    Act_Thresh_Min = 1
    Desired_Pace = LRL
  state SETACTLVL
    entry:
    Act_Lvl = Accel*1.35
    m_slope=(MSR-LRL)/(Act_Thresh_Max-Act_Thresh_Min);
  state check3
    entry:
    Desired_Pace = MSR
  SETACTLVL -> SETACTLVL [order 2] : [Act_Lvl<=Act_Thresh]
  check -> check2 [order 1] : [Desired_Pace1<MSR]
  SETACTLVL -> check [order 1] : [Act_Lvl> Act_Thresh]
  check2 -> (junction 96)
  check -> check3 [order 2] : [Desired_Pace1>=MSR]
  (default) -> init
  init -> SETACTLVL
  check3 -> (junction 96)
  (junction 96) -> SETACTLVL
  data: Act_Thresh input double; RF input double; Desired_Pace output double; Accel input double; Act_Lvl local; Act_Thresh_Max local; Act_Thresh_Min local; m_slope local; LRL input; MSR input; Desired_Pace1 local

== stateflow chart assignment2_group12/big Subsystem/Chart ==
  state SET_PARAMETERS
    entry:
    mode=rxdata(3);
    LRL=typecast(rxdata(4:11),'double');
    URL=typecast(rxdata(12:19),'double');
    Atr_Amp=typecast(rxdata(20:27),'double');
    Atr_Pul_Wid=typecast(rxdata(28:35),'double');
    Atr_Sen= typecast(rxdata(36:43),'double');
    ARP=typecast(rxdata(44:51),'double');
    Ven_Amp=typecast(rxdata(52:59),'double');
    Ven_Pul_Wid=typecast(rxdata(60:67),'double');
    Ven_Sen=typecast(rxdata(68:75),'double');
    VRP=typecast(rxdata(76:83),'double');
    MSR=typecast(rxdata(84:91),'double');
    Act_Thresh=typecast(rxdata(92:99),'double');
    Rxn_Time=typecast(rxdata(100:107),'double');
    RF=typecast(rxdata(108:115),'double');
    Rec_Time=typecast(rxdata(116:123),'double');
  state NOMINAL_VALUES
    entry:
    mode=1;
    LRL=60;
    URL=120;
    Atr_Amp=5.0;
    Atr_Pul_Wid=1;
    Atr_Sen=.75;
    ARP=250;
    Ven_Amp=5.0;
    Ven_Pul_Wid=1;
    Ven_Sen=2.5;
    VRP=250;
    MSR=120;
    Act_Thresh= 4;
    Rxn_Time=30;
    RF=8;
    Rec_Time=5
  state STANDBY
  state ECHO_PARAM
    entry:
    %Send Values to DCM
    send_back()
  SET_PARAMETERS -> STANDBY
  (junction 10) -> SET_PARAMETERS [order 1] : [rxdata(2)==hex2dec('22')]
  (default) -> NOMINAL_VALUES
  STANDBY -> (junction 10) : [rxdata(1) == hex2dec('16')]
  NOMINAL_VALUES -> STANDBY
  (junction 10) -> ECHO_PARAM [order 2] : [rxdata(2) == hex2dec('55')]
  ECHO_PARAM -> STANDBY
  data: rxdata input uint8; LRL output double; Atr_Amp output double; URL output double; Atr_Pul_Wid output double; Atr_Sen output double; ARP output double; Ven_Amp output double; Ven_Pul_Wid output double; Ven_Sen output double; VRP output double; MSR output double; Act_Thresh output double; Rxn_Time output double; RF output double; Rec_Time output double; mode output uint8
  events: send_params local RISING_EDGE_EVENT

== stateflow chart assignment2_group12/big Subsystem/Subsystem/Rate Adaptive ==
  state check
  state TIME_UP
    entry:
    Time_Up= ((Desired_Pace-Current_Pace)*Rxn_Time*1000)/(MSR-LRL)
    Increment=(Desired_Pace-Current_Pace)/Time_Up
    Current_Pace = Current_Pace + Increment
  state START
    Current_Pace=LRL
  state TIME_DOWN
    entry:
    Time_Down=((Desired_Pace-Current_Pace)*Rec_Time*60000)/(MSR-LRL)
    Decrement=(Desired_Pace-Current_Pace)/Time_Down
    Current_Pace = Current_Pace + Decrement
  TIME_UP -> check
  START -> check
  check -> TIME_UP [order 2] : [Desired_Pace>Current_Pace]
  (default) -> START
  check -> TIME_DOWN [order 1] : [Desired_Pace<Current_Pace]
  TIME_DOWN -> check
  data: Desired_Pace input double; Current_Pace output double; LRL input; MSR input; Rxn_Time input; Rec_Time input; Time_Down local; Increment local; Time_Up local; Timing local; Decrement local
